simulink model "Problem4"  (R2020b)
settings: Solver=VariableStepAuto  StartTime=0.0  StopTime=10.0  RelTol=1e-3
model workspace (MAT data in the model file):
  x = Simulink.Parameter
  x.Value = 1
  x.DataType = 'auto'
  x.Dimensions = [1 1]
settings Model: Creator=admin  LastModifiedBy=admin

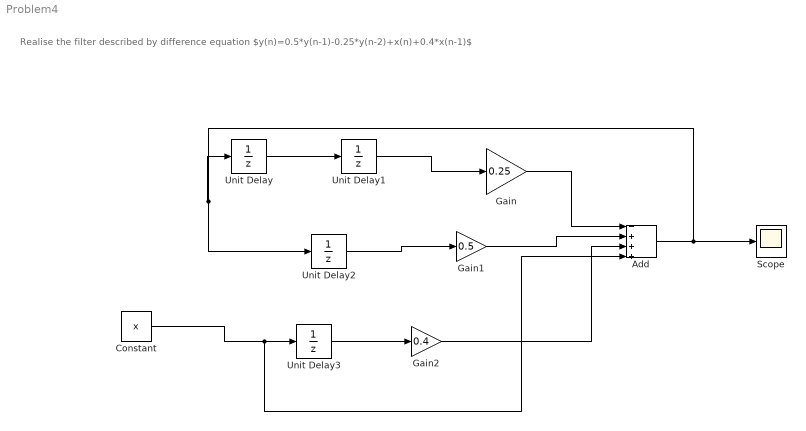
== system Problem4 ==
  note: Realise the filter described by difference equation
      | $y(n)=0.5*y(n-1)-0.25*y(n-2)+x(n)+0.4*x(n-1)$
  Add : Sum  Inputs=-+++
  Constant : Constant  Value=x
  Gain : Gain  Gain=0.25
  Gain1 : Gain  Gain=0.5
  Gain2 : Gain  Gain=0.4
  Scope : Scope
  Unit Delay{,1..3} (4 alike) : UnitDelay  SampleTime=-1  HasFrameUpgradeWarning=on
  wires:
  Gain/1 -> Add/1
  Gain1/1 -> Add/2
  Gain2/1 -> Add/3
  Unit Delay2/1 -> Gain1/1
  Unit Delay1/1 -> Gain/1
  Unit Delay/1 -> Unit Delay1/1
  Add/1 -> Unit Delay2/1, Unit Delay/1, Scope/1
  Unit Delay3/1 -> Gain2/1
  Constant/1 -> Add/4, Unit Delay3/1
